simulink model "CalcTimes"  (R2024b)
settings: Solver=VariableStepAuto  StartTime=0.0  StopTime=10.0  RelTol=1e-3
settings Model: Creator=ryandavis  LastModifiedBy=ryandavis

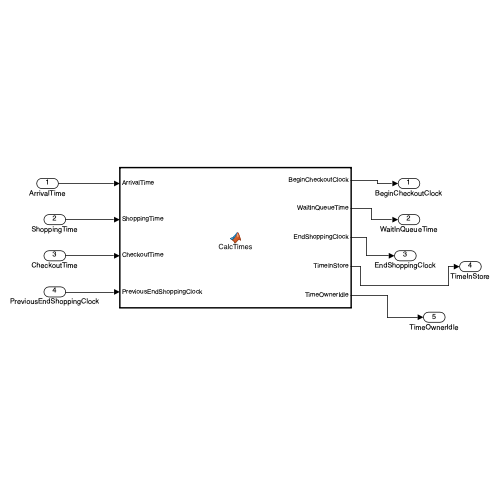
[thumbnail: Simulink's stored preview of the top-level diagram]
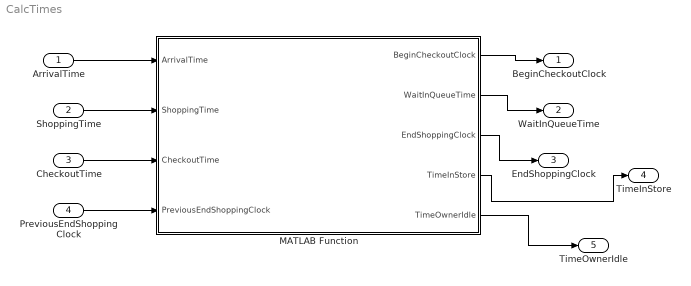
== system CalcTimes ==
  ArrivalTime : Inport
  ShoppingTime : Inport  Port=2
  CheckoutTime : Inport  Port=3
  PreviousEndShoppingClock : Inport  Port=4
  MATLAB Function : MATLAB Function  TreatAsAtomicUnit=on
  BeginCheckoutClock : Outport
  WaitInQueueTime : Outport  Port=2
  EndShoppingClock : Outport  Port=3
  TimeInStore : Outport  Port=4
  TimeOwnerIdle : Outport  Port=5
  wires:
  CheckoutTime/1 -> MATLAB Function/3(CheckoutTime)
  ShoppingTime/1 -> MATLAB Function/2(ShoppingTime)
  ArrivalTime/1 -> MATLAB Function/1(ArrivalTime)
  PreviousEndShoppingClock/1 -> MATLAB Function/4(PreviousEndShoppingClock)
  MATLAB Function/1(BeginCheckoutClock) -> BeginCheckoutClock/1
  MATLAB Function/2(WaitInQueueTime) -> WaitInQueueTime/1
  MATLAB Function/3(EndShoppingClock) -> EndShoppingClock/1
  MATLAB Function/4(TimeInStore) -> TimeInStore/1
  MATLAB Function/5(TimeOwnerIdle) -> TimeOwnerIdle/1

== matlab function CalcTimes/MATLAB Function ==
  data: ArrivalTime input; BeginCheckoutClock output; ShoppingTime input; CheckoutTime input; PreviousEndShoppingClock input; WaitInQueueTime output; EndShoppingClock output; TimeInStore output; TimeOwnerIdle output
function [BeginCheckoutClock, WaitInQueueTime, EndShoppingClock, TimeInStore, TimeOwnerIdle] = CalcTimes(ArrivalTime, ShoppingTime, CheckoutTime, PreviousEndShoppingClock)
    BeginCheckoutClock = ArrivalTime + ShoppingTime;
    
    WaitInQueueTime = max(0, PreviousEndShoppingClock - BeginCheckoutClock);
    
    EndShoppingClock = BeginCheckoutClock + WaitInQueueTime + CheckoutTime;
    
    TimeInStore = EndShoppingClock - ArrivalTime;
    
    TimeOwnerIdle = max(0, BeginCheckoutClock - PreviousEndShoppingClock);
end
